simulink model "SF015A_WhlImbRejctn"  (R2013b)
settings: Solver=FixedStepDiscrete  SolverMode=SingleTasking  StartTime=0.0  StopTime=1  FixedStep=0.002  RelTol=1e-3
values from neighbouring files (symbols this model uses):
  ACTIVBANDMAX_ULS_U32 = DataDict.Constant    [SF015A_WhlImbRejctn_DataDict.m]
  ADAPVFILMAX_ULS_F32 = DataDict.Constant    [SF015A_WhlImbRejctn_DataDict.m]
  ARCHGLBPRM_180OVERPI_ULS_F32 = DataDict.Constant    [SF015A_WhlImbRejctn_DataDict.m]
  ARCHGLBPRM_2MILLISEC_SEC_F32 = DataDict.Constant    [SF015A_WhlImbRejctn_DataDict.m]
  ARCHGLBPRM_2PI_ULS_F32 = DataDict.Constant    [SF015A_WhlImbRejctn_DataDict.m]
  ARCHGLBPRM_FLOATZEROTHD_ULS_F32 = DataDict.Constant    [SF015A_WhlImbRejctn_DataDict.m]
  ARCHGLBPRM_PI_ULS_F32 = DataDict.Constant    [SF015A_WhlImbRejctn_DataDict.m]
  ARCHGLBPRM_PIOVER180_ULS_F32 = DataDict.Constant    [SF015A_WhlImbRejctn_DataDict.m]
  ARCHGLBPRM_PIOVER2_ULS_F32 = DataDict.Constant    [SF015A_WhlImbRejctn_DataDict.m]
  CALMINSPERCOUNT_ULS_F32 = DataDict.Constant    [SF015A_WhlImbRejctn_DataDict.m]
  DURATIONDISABLE_CNT_U16 = DataDict.Constant    [SF015A_WhlImbRejctn_DataDict.m]
  FILTWHLSPDMAX_MOTRADPERSEC_F32 = DataDict.Constant    [SF015A_WhlImbRejctn_DataDict.m]
  MICROSECTOMILLISEC_ULS_F32 = DataDict.Constant    [SF015A_WhlImbRejctn_DataDict.m]
  MINSTOMILLISEC_ULS_F32 = DataDict.Constant    [SF015A_WhlImbRejctn_DataDict.m]
  NINETY_ULS_F32 = DataDict.Constant    [SF015A_WhlImbRejctn_DataDict.m]
  NODEBSTEP_CNT_U16 = DataDict.Constant    [SF015A_WhlImbRejctn_DataDict.m]
  NROFDLY_CNT_U08 = DataDict.Constant    [SF015A_WhlImbRejctn_DataDict.m]
  ONEHALF_ULS_F32 = DataDict.Constant    [SF015A_WhlImbRejctn_DataDict.m]
  ONEHUNDRED_ULS_F32 = DataDict.Constant    [SF015A_WhlImbRejctn_DataDict.m]
  ONEOVRTHREE_ULS_F32 = DataDict.Constant    [SF015A_WhlImbRejctn_DataDict.m]
  ONEOVRTWENTY_ULS_F32 = DataDict.Constant    [SF015A_WhlImbRejctn_DataDict.m]
  ONETHOUSAND_ULS_F32 = DataDict.Constant    [SF015A_WhlImbRejctn_DataDict.m]
  PEAKMAX_ULS_F32 = DataDict.Constant    [SF015A_WhlImbRejctn_DataDict.m]
  PEAKMIN_ULS_F32 = DataDict.Constant    [SF015A_WhlImbRejctn_DataDict.m]
  PHAADJMAX_ULS_F32 = DataDict.Constant    [SF015A_WhlImbRejctn_DataDict.m]
  PITIMESSAMPLETIME_ULS_F32 = DataDict.Constant    [SF015A_WhlImbRejctn_DataDict.m]
  STOREDMINSPERCOUNT_ULS_F32 = DataDict.Constant    [SF015A_WhlImbRejctn_DataDict.m]
  TWO_ULS_F32 = DataDict.Constant    [SF015A_WhlImbRejctn_DataDict.m]
  TWOOVRTHREE_ULS_F32 = DataDict.Constant    [SF015A_WhlImbRejctn_DataDict.m]
  WhlImbRejctnAdpvFac = DataDict.Calibration    [SF015A_WhlImbRejctn_DataDict.m]
  WhlImbRejctnAutScaEna = DataDict.Calibration    [SF015A_WhlImbRejctn_DataDict.m]
  WhlImbRejctnAutScaTar = DataDict.Calibration    [SF015A_WhlImbRejctn_DataDict.m]
  WhlImbRejctnCurrMgnSlewPerLoop = DataDict.Calibration    [SF015A_WhlImbRejctn_DataDict.m]
  WhlImbRejctnDcTrendFltRcvryDly = DataDict.Calibration    [SF015A_WhlImbRejctn_DataDict.m]
  WhlImbRejctnDcTrendFltRcvryNegStep = DataDict.Calibration    [SF015A_WhlImbRejctn_DataDict.m]
  WhlImbRejctnDcTrendFltRcvryPosStep = DataDict.Calibration    [SF015A_WhlImbRejctn_DataDict.m]
  WhlImbRejctnDcTrendFltRcvryThd = DataDict.Calibration    [SF015A_WhlImbRejctn_DataDict.m]
  WhlImbRejctnDcTrendTh2Tq = DataDict.Calibration    [SF015A_WhlImbRejctn_DataDict.m]
  WhlImbRejctnDcTrendThTq = DataDict.Calibration    [SF015A_WhlImbRejctn_DataDict.m]
  WhlImbRejctnDcTrendTi2Sec = DataDict.Calibration    [SF015A_WhlImbRejctn_DataDict.m]
  WhlImbRejctnDcTrendTiSec = DataDict.Calibration    [SF015A_WhlImbRejctn_DataDict.m]
  WhlImbRejctnEnaSlewPerLoop = DataDict.Calibration    [SF015A_WhlImbRejctn_DataDict.m]
  WhlImbRejctnFctEna = DataDict.Calibration    [SF015A_WhlImbRejctn_DataDict.m]
  WhlImbRejctnFrqDiagcAmpThd = DataDict.Calibration    [SF015A_WhlImbRejctn_DataDict.m]
  WhlImbRejctnFrqDiagcEna = DataDict.Calibration    [SF015A_WhlImbRejctn_DataDict.m]
  WhlImbRejctnFrqDiagcFltRcvryDly = DataDict.Calibration    [SF015A_WhlImbRejctn_DataDict.m]
  WhlImbRejctnFrqDiagcFltRcvryNegStep = DataDict.Calibration    [SF015A_WhlImbRejctn_DataDict.m]
  WhlImbRejctnFrqDiagcFltRcvryPosStep = DataDict.Calibration    [SF015A_WhlImbRejctn_DataDict.m]
  WhlImbRejctnFrqDiagcFltRcvryThd = DataDict.Calibration    [SF015A_WhlImbRejctn_DataDict.m]
  WhlImbRejctnFrqDiagcThd = DataDict.Calibration    [SF015A_WhlImbRejctn_DataDict.m]
  WhlImbRejctnFrqDiagcTout = DataDict.Calibration    [SF015A_WhlImbRejctn_DataDict.m]
  WhlImbRejctnFrqDiagcUgrPoleMgn = DataDict.Calibration    [SF015A_WhlImbRejctn_DataDict.m]
  WhlImbRejctnFrqScaTblX = DataDict.Calibration    [SF015A_WhlImbRejctn_DataDict.m]
  WhlImbRejctnMaxDurn = DataDict.Calibration    [SF015A_WhlImbRejctn_DataDict.m]
  WhlImbRejctnMaxMgn = DataDict.Calibration    [SF015A_WhlImbRejctn_DataDict.m]
  WhlImbRejctnMaxMgnFltNegStep = DataDict.Calibration    [SF015A_WhlImbRejctn_DataDict.m]
  WhlImbRejctnMaxMgnFltPosStep = DataDict.Calibration    [SF015A_WhlImbRejctn_DataDict.m]
  WhlImbRejctnMaxMgnFltRcvryDly = DataDict.Calibration    [SF015A_WhlImbRejctn_DataDict.m]
  WhlImbRejctnMaxMgnFltRcvryNegStep = DataDict.Calibration    [SF015A_WhlImbRejctn_DataDict.m]
  WhlImbRejctnMaxMgnFltRcvryPosStep = DataDict.Calibration    [SF015A_WhlImbRejctn_DataDict.m]
  WhlImbRejctnMaxMgnFltRcvryThd = DataDict.Calibration    [SF015A_WhlImbRejctn_DataDict.m]
  WhlImbRejctnMaxMgnFltThd = DataDict.Calibration    [SF015A_WhlImbRejctn_DataDict.m]
  WhlImbRejctnMgnEstimnDeltaSca = DataDict.Calibration    [SF015A_WhlImbRejctn_DataDict.m]
  WhlImbRejctnMgnEstimnDiThd = DataDict.Calibration    [SF015A_WhlImbRejctn_DataDict.m]
  WhlImbRejctnMgnEstimnEnaThd = DataDict.Calibration    [SF015A_WhlImbRejctn_DataDict.m]
  WhlImbRejctnMgnEstimnFrq = DataDict.Calibration    [SF015A_WhlImbRejctn_DataDict.m]
  WhlImbRejctnMgnEstimnFrqDelta = DataDict.Calibration    [SF015A_WhlImbRejctn_DataDict.m]
  WhlImbRejctnMgnEstimnLeak = DataDict.Calibration    [SF015A_WhlImbRejctn_DataDict.m]
  WhlImbRejctnRampDwnTi = DataDict.Calibration    [SF015A_WhlImbRejctn_DataDict.m]
  WhlImbRejctnScaCncl = DataDict.Calibration    [SF015A_WhlImbRejctn_DataDict.m]
  WhlImbRejctnUgrPoleMgn = DataDict.Calibration    [SF015A_WhlImbRejctn_DataDict.m]
  WhlImbRejctnVehSpdEna = DataDict.Calibration    [SF015A_WhlImbRejctn_DataDict.m]
  WhlImbRejctnWhlSpdCorrlnFltRcvryDly = DataDict.Calibration    [SF015A_WhlImbRejctn_DataDict.m]
  WhlImbRejctnWhlSpdCorrlnFltRcvryNegStep = DataDict.Calibration    [SF015A_WhlImbRejctn_DataDict.m]
  WhlImbRejctnWhlSpdCorrlnFltRcvryPosStep = DataDict.Calibration    [SF015A_WhlImbRejctn_DataDict.m]
  WhlImbRejctnWhlSpdCorrlnFltRcvryThd = DataDict.Calibration    [SF015A_WhlImbRejctn_DataDict.m]
  WhlImbRejctnWhlSpdCorrlnThd = DataDict.Calibration    [SF015A_WhlImbRejctn_DataDict.m]
  WhlImbRejctnWhlSpdCorrlnTi = DataDict.Calibration    [SF015A_WhlImbRejctn_DataDict.m]
  WIRCMDMAX_MOTNWTMTR_F32 = DataDict.Constant    [SF015A_WhlImbRejctn_DataDict.m]
  ZERO_ULS_F32 = DataDict.Constant    [SF015A_WhlImbRejctn_DataDict.m]
undefined symbols (not defined in the file or in its folder): Cntr, NtcNr1, NvmGetErrSts1, SigQlfr1, Sts, SysSt1
libraries: simulink x32, FixdToFloat x32, Fil x20, NxtrLim x15, NxtrNvM x12, NxtrAbslt x8, NxtrMath x7, NxtrMax x6, NxtrMin x4, FloatToFixd x2, LnrIntrpn x2, NxtrSign x1
(part 3 of 12)

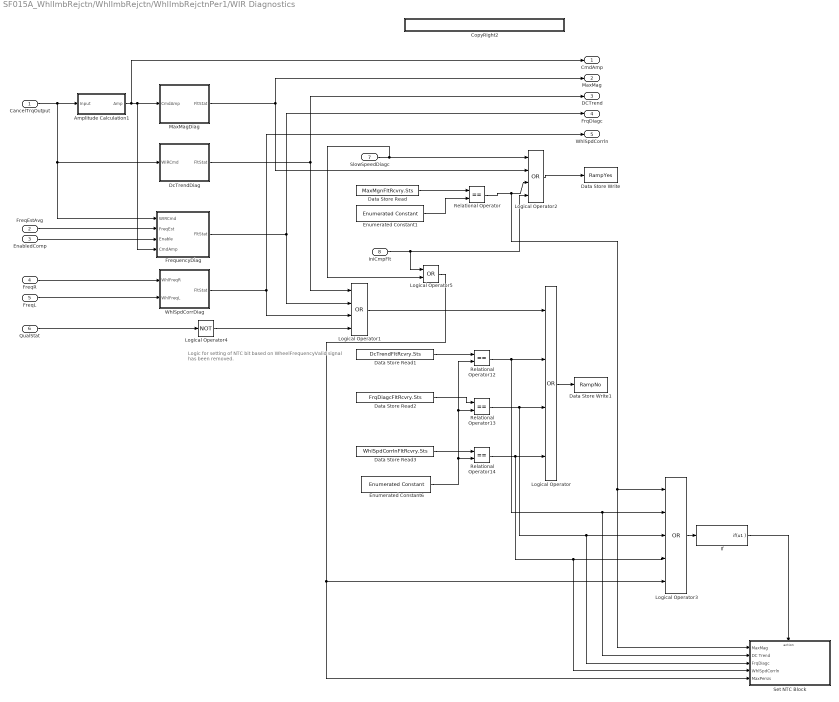
== system SF015A_WhlImbRejctn/WhlImbRejctn/WhlImbRejctnPer1/WIR Diagnostics ==
  note: Logic for setting of NTC bit based on WheelFrequencyValid
      | signal has been removed.
  CancelTrqOutput : Inport
  FreqEstAvg : Inport  Port=2
  EnabledComp : Inport  Port=3
  FreqR : Inport  Port=4
  FreqL : Inport  Port=5
  QualStat : Inport  Port=6
  "SlowSpeedDiagc " : Inport  Port=7
  IniCmpFlt : Inport  Port=8
  Amplitude Calculation1 : Subsystem
  CopyRight2 : Subsystem  Description=|  mask(Copyright Information){none=on}
      | Copyright info block.                                               
      |                                                                     
      | Place copyright information at the top of every subsystem in design.
      mask prompts: none "No parameters"
      mask help: Place copyright information at the top of every subsystem in design.
      mask Display:
      | NxtrConf = 'Nexteer Confidential';
      | 
      | sys = bdroot; %handle for the current model ("system")
      | first = get_param(sys,'Created');
      | first = first(end-3:end);  %year is last four digits
      | 
      | last = get_param(sys,'LastModifiedDate');
      | if isempty(last)
      |     last = datestr(now,'yyyy');
      | else
      |     last = last(end-3:end);
      | end
      | 
      | if strcmp(first,last)
      |     fprintf('%s -- Copyright %s Nexteer',NxtrConf,first)
      | else
      |     fprintf('%s -- %s%s- %s Nexteer',NxtrConf,char(169),first,last)
      | end
  Data Store Read : DataStoreRead  DataStoreName=MaxMgnFltRcvry  DataStoreElements=MaxMgnFltRcvry.Sts
  Data Store Read1 : DataStoreRead  DataStoreName=DcTrendFltRcvry  DataStoreElements=DcTrendFltRcvry.Sts
  Data Store Read2 : DataStoreRead  DataStoreName=FrqDiagcFltRcvry  DataStoreElements=FrqDiagcFltRcvry.Sts
  Data Store Read3 : DataStoreRead  DataStoreName=WhlSpdCorrlnFltRcvry  DataStoreElements=WhlSpdCorrlnFltRcvry.Sts
  Data Store Write : DataStoreWrite  DataStoreName=RampYes
  Data Store Write1 : DataStoreWrite  DataStoreName=RampNo
  DcTrendDiag : Subsystem
  Enumerated Constant1 : simulink/Sources/Enumerated Constant  OutDataTypeStr=Enum: SigQlfr1  Value=SigQlfr1.SIGQLFR_FAILD  SampleTime=inf
  Enumerated Constant6 : simulink/Sources/Enumerated Constant  OutDataTypeStr=Enum: SigQlfr1  Value=SigQlfr1.SIGQLFR_FAILD  SampleTime=inf
  FrequencyDiag : Subsystem
  If : If  IfExpression=u1  ShowElse=off
  Logical Operator : Logic  Operator=OR  Inputs=4  AllPortsSameDT=off  OutDataTypeStr=boolean
  Logical Operator1 : Logic  Operator=OR  Inputs=4  AllPortsSameDT=off  OutDataTypeStr=boolean
  Logical Operator2 : Logic  Operator=OR  Inputs=4  AllPortsSameDT=off  OutDataTypeStr=boolean
  Logical Operator3 : Logic  Operator=OR  Inputs=5  AllPortsSameDT=off  OutDataTypeStr=boolean
  Logical Operator4 : Logic  Operator=NOT  AllPortsSameDT=off  OutDataTypeStr=boolean
  Logical Operator5 : Logic  Operator=OR  AllPortsSameDT=off  OutDataTypeStr=boolean
  MaxMagDiag : Subsystem
  Relational Operator{,12..14} (4 alike) : RelationalOperator  Operator===  OutDataTypeStr=boolean
  Set NTC Block : Subsystem  TreatAsAtomicUnit=on
  WhlSpdCorrDiag : Subsystem
  CmdAmp : Outport
  MaxMag : Outport  Port=2
  DCTrend : Outport  Port=3
  FrqDiagc : Outport  Port=4
  WhlSpdCorrln : Outport  Port=5
  wires:
  CancelTrqOutput/1 -> Amplitude Calculation1/1(Input), FrequencyDiag/1(WIRCmd), DcTrendDiag/1(WIRCmd)
  EnabledComp/1 -> FrequencyDiag/3(Enable)
  FreqEstAvg/1 -> FrequencyDiag/2(FreqEst)
  FreqR/1 -> WhlSpdCorrDiag/1(WhlFreqR)
  FreqL/1 -> WhlSpdCorrDiag/2(WhlFreqL)
  DcTrendDiag/1(FltStat) -> DCTrend/1, Logical Operator1/1
  MaxMagDiag/1(FltStat) -> MaxMag/1, Logical Operator2/2
  FrequencyDiag/1(FltStat) -> FrqDiagc/1, Logical Operator1/2
  WhlSpdCorrDiag/1(FltStat) -> WhlSpdCorrln/1, Logical Operator1/3
  Amplitude Calculation1/1(Amp) -> CmdAmp/1, MaxMagDiag/1(CmdAmp), FrequencyDiag/4(CmdAmp)
  Relational Operator12/1 -> Logical Operator/2, Set NTC Block/2(DC Trend), Logical Operator3/2
  Relational Operator14/1 -> Logical Operator3/4, Set NTC Block/4(WhlSpdCorrln), Logical Operator/4
  Enumerated Constant6/1 -> Relational Operator12/2, Relational Operator13/2, Relational Operator14/2
  Logical Operator1/1 -> Logical Operator/1
  Logical Operator2/1 -> Data Store Write/1
  "SlowSpeedDiagc "/1 -> Logical Operator5/2, Logical Operator2/1
  Data Store Read/1 -> Relational Operator/1
  Enumerated Constant1/1 -> Relational Operator/2
  Relational Operator/1 -> Set NTC Block/1(MaxMag), Logical Operator3/1, Logical Operator2/3
  Data Store Read1/1 -> Relational Operator12/1
  Data Store Read3/1 -> Relational Operator14/1
  Data Store Read2/1 -> Relational Operator13/1
  Logical Operator3/1 -> If/1
  If/1 -> Set NTC Block/Action
  Logical Operator/1 -> Data Store Write1/1
  Relational Operator13/1 -> Logical Operator3/3, Set NTC Block/3(FrqDiagc), Logical Operator/3
  QualStat/1 -> Logical Operator4/1
  Logical Operator4/1 -> Logical Operator1/4
  IniCmpFlt/1 -> Logical Operator5/1, Logical Operator2/4
  Logical Operator5/1 -> Logical Operator3/5, Set NTC Block/5(MaxPersis)

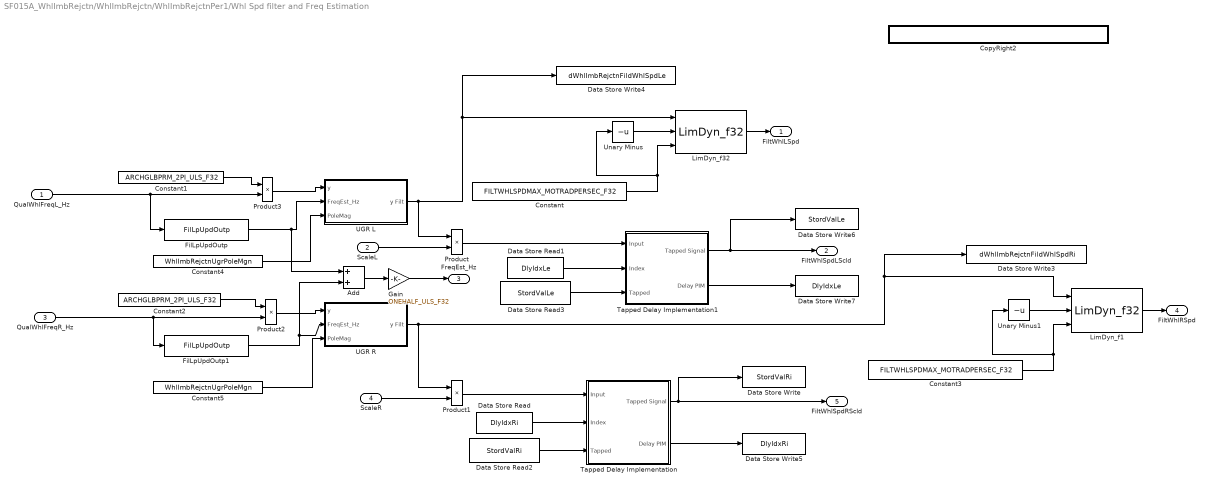
== system SF015A_WhlImbRejctn/WhlImbRejctn/WhlImbRejctnPer1/Whl Spd filter and Freq Estimation ==
  QualWhlFreqL_Hz : Inport
  ScaleL : Inport  Port=2
  QualWhlFreqR_Hz : Inport  Port=3
  ScaleR : Inport  Port=4
  Add : Sum
  Constant : Constant  Value=FILTWHLSPDMAX_MOTRADPERSEC_F32
  Constant1 : Constant  Value=ARCHGLBPRM_2PI_ULS_F32
  Constant2 : Constant  Value=ARCHGLBPRM_2PI_ULS_F32
  Constant3 : Constant  Value=FILTWHLSPDMAX_MOTRADPERSEC_F32
  Constant4 : Constant  Value=WhlImbRejctnUgrPoleMgn
  Constant5 : Constant  Value=WhlImbRejctnUgrPoleMgn
  CopyRight2 : Subsystem  Description=|  mask(Copyright Information){none=on}
      | Copyright info block.                                               
      |                                                                     
      | Place copyright information at the top of every subsystem in design.
      mask prompts: none "No parameters"
      mask help: Place copyright information at the top of every subsystem in design.
      mask Display:
      | NxtrConf = 'Nexteer Confidential';
      | 
      | sys = bdroot; %handle for the current model ("system")
      | first = get_param(sys,'Created');
      | first = first(end-3:end);  %year is last four digits
      | 
      | last = get_param(sys,'LastModifiedDate');
      | if isempty(last)
      |     last = datestr(now,'yyyy');
      | else
      |     last = last(end-3:end);
      | end
      | 
      | if strcmp(first,last)
      |     fprintf('%s -- Copyright %s Nexteer',NxtrConf,first)
      | else
      |     fprintf('%s -- %s%s- %s Nexteer',NxtrConf,char(169),first,last)
      | end
  Data Store Read : DataStoreRead  DataStoreName=DlyIdxRi
  Data Store Read1 : DataStoreRead  DataStoreName=DlyIdxLe
  Data Store Read2 : DataStoreRead  DataStoreName=StordValRi
  Data Store Read3 : DataStoreRead  DataStoreName=StordValLe
  Data Store Write : DataStoreWrite  DataStoreName=StordValRi
  Data Store Write3 : DataStoreWrite  DataStoreName=dWhlImbRejctnFildWhlSpdRi
  Data Store Write4 : DataStoreWrite  DataStoreName=dWhlImbRejctnFildWhlSpdLe
  Data Store Write5 : DataStoreWrite  DataStoreName=DlyIdxRi
  Data Store Write6 : DataStoreWrite  DataStoreName=StordValLe
  Data Store Write7 : DataStoreWrite  DataStoreName=DlyIdxLe
  FilLpUpdOutp : Fil/FilLpUpdOutp  StVar=WhlSpdLeLpFil
      settings: AttributesFormatString=StVar: %<StVar>
  FilLpUpdOutp1 : Fil/FilLpUpdOutp  StVar=WhlSpdRiLpFil
      settings: AttributesFormatString=StVar: %<StVar>
  Gain : Gain  Gain=ONEHALF_ULS_F32
  LimDyn_f1 : NxtrLim/LimDyn_f32
  LimDyn_f32 : NxtrLim/LimDyn_f32
  Product{,1..3} (4 alike) : Product
  Tapped Delay Implementation : Subsystem  TreatAsAtomicUnit=on
  Tapped Delay Implementation1 : Subsystem  TreatAsAtomicUnit=on
  UGR L : Subsystem
  UGR R : Subsystem
  Unary Minus : UnaryMinus
  Unary Minus1 : UnaryMinus
  FiltWhlLSpd : Outport
  FiltWhlSpdLScld : Outport  Port=2
  FreqEst_Hz : Outport  Port=3
  FiltWhlRSpd : Outport  Port=4
  FiltWhlSpdRScld : Outport  Port=5
  wires:
  UGR L/1(y Filt) -> Product/1, LimDyn_f32/1, Data Store Write4/1
  FilLpUpdOutp/1 -> Add/1, UGR L/2(FreqEst_Hz)
  QualWhlFreqL_Hz/1 -> FilLpUpdOutp/1, Product3/2
  Product/1 -> Tapped Delay Implementation1/1(Input)
  ScaleL/1 -> Product/2
  Constant1/1 -> Product3/1
  Product3/1 -> UGR L/1(y)
  UGR R/1(y Filt) -> Product1/1, Data Store Write3/1, LimDyn_f1/1
  FilLpUpdOutp1/1 -> UGR R/2(FreqEst_Hz), Add/2
  QualWhlFreqR_Hz/1 -> FilLpUpdOutp1/1, Product2/2
  Product1/1 -> Tapped Delay Implementation/1(Input)
  Constant2/1 -> Product2/1
  Product2/1 -> UGR R/1(y)
  ScaleR/1 -> Product1/2
  Add/1 -> Gain/1
  Gain/1 -> FreqEst_Hz/1
  Data Store Read/1 -> Tapped Delay Implementation/2(Index)
  Data Store Read2/1 -> Tapped Delay Implementation/3(Tapped)
  Tapped Delay Implementation/1(Tapped Signal) -> Data Store Write/1, FiltWhlSpdRScld/1
  Tapped Delay Implementation/2(Delay PIM) -> Data Store Write5/1
  Tapped Delay Implementation1/1(Tapped Signal) -> Data Store Write6/1, FiltWhlSpdLScld/1
  Tapped Delay Implementation1/2(Delay PIM) -> Data Store Write7/1
  Data Store Read1/1 -> Tapped Delay Implementation1/2(Index)
  Data Store Read3/1 -> Tapped Delay Implementation1/3(Tapped)
  LimDyn_f32/1 -> FiltWhlLSpd/1
  Constant/1 -> Unary Minus/1, LimDyn_f32/3
  Unary Minus/1 -> LimDyn_f32/2
  LimDyn_f1/1 -> FiltWhlRSpd/1
  Constant3/1 -> Unary Minus1/1, LimDyn_f1/3
  Unary Minus1/1 -> LimDyn_f1/2
  Constant4/1 -> UGR L/3(PoleMag)
  Constant5/1 -> UGR R/3(PoleMag)

== system SF015A_WhlImbRejctn/WhlImbRejctn/WhlImbRejctnPer2/CopyRight2 ==

== system SF015A_WhlImbRejctn/WhlImbRejctn/WhlImbRejctnPer2/Flt Recovery- DC Trend ==
  FltStatIn : Inport
  FltRecDly : Inport  Port=2
  Constant : Constant  Value=MINSTOMILLISEC_ULS_F32
  CopyRight2 : Subsystem  Description=|  mask(Copyright Information){none=on}
      | Copyright info block.                                               
      |                                                                     
      | Place copyright information at the top of every subsystem in design.
      mask prompts: none "No parameters"
      mask help: Place copyright information at the top of every subsystem in design.
      mask Display:
      | NxtrConf = 'Nexteer Confidential';
      | 
      | sys = bdroot; %handle for the current model ("system")
      | first = get_param(sys,'Created');
      | first = first(end-3:end);  %year is last four digits
      | 
      | last = get_param(sys,'LastModifiedDate');
      | if isempty(last)
      |     last = datestr(now,'yyyy');
      | else
      |     last = last(end-3:end);
      | end
      | 
      | if strcmp(first,last)
      |     fprintf('%s -- Copyright %s Nexteer',NxtrConf,first)
      | else
      |     fprintf('%s -- %s%s- %s Nexteer',NxtrConf,char(169),first,last)
      | end
  Data Store Read : DataStoreRead  Priority=1  DataStoreName=DcTrendFltRcvry
      settings: AttributesFormatString=Priority:%<Priority>
  Data Store Write1 : DataStoreWrite  Priority=2  DataStoreName=DcTrendFltRcvry
      settings: AttributesFormatString=Priority:%<Priority>
  Divide : Product  Inputs=**
  ElapsedTime1 : Subsystem  TreatAsAtomicUnit=on
  Relational Operator4 : RelationalOperator  OutDataTypeStr=boolean
  Update Fault Status : Subsystem  TreatAsAtomicUnit=on
  wires:
  ElapsedTime1/1(ElapsedTime) -> Relational Operator4/1
  FltStatIn/1 -> ElapsedTime1/1(FltStsTrue)
  FltRecDly/1 -> Divide/1
  Relational Operator4/1 -> Update Fault Status/2(Status)
  Data Store Read/1 -> Update Fault Status/1(Structvar)
  Update Fault Status/1(Structvar_out) -> Data Store Write1/1
  Divide/1 -> Relational Operator4/2
  Constant/1 -> Divide/2

== system SF015A_WhlImbRejctn/WhlImbRejctn/WhlImbRejctnPer2/Flt Recovery- Freq Diag ==
  FltStatIn : Inport
  FltRecDly : Inport  Port=2
  Constant : Constant  Value=MINSTOMILLISEC_ULS_F32
  CopyRight2 : Subsystem  Description=|  mask(Copyright Information){none=on}
      | Copyright info block.                                               
      |                                                                     
      | Place copyright information at the top of every subsystem in design.
      mask prompts: none "No parameters"
      mask help: Place copyright information at the top of every subsystem in design.
      mask Display:
      | NxtrConf = 'Nexteer Confidential';
      | 
      | sys = bdroot; %handle for the current model ("system")
      | first = get_param(sys,'Created');
      | first = first(end-3:end);  %year is last four digits
      | 
      | last = get_param(sys,'LastModifiedDate');
      | if isempty(last)
      |     last = datestr(now,'yyyy');
      | else
      |     last = last(end-3:end);
      | end
      | 
      | if strcmp(first,last)
      |     fprintf('%s -- Copyright %s Nexteer',NxtrConf,first)
      | else
      |     fprintf('%s -- %s%s- %s Nexteer',NxtrConf,char(169),first,last)
      | end
  Data Store Read : DataStoreRead  Priority=1  DataStoreName=FrqDiagcFltRcvry
      settings: AttributesFormatString=Priority:%<Priority>
  Data Store Write1 : DataStoreWrite  Priority=2  DataStoreName=FrqDiagcFltRcvry
      settings: AttributesFormatString=Priority:%<Priority>
  Divide : Product  Inputs=**
  ElapsedTime1 : Subsystem  TreatAsAtomicUnit=on
  Relational Operator4 : RelationalOperator  OutDataTypeStr=boolean
  Update Fault Status : Subsystem  TreatAsAtomicUnit=on
  wires:
  ElapsedTime1/1(ElapsedTime) -> Relational Operator4/1
  FltStatIn/1 -> ElapsedTime1/1(FltStsTrue)
  FltRecDly/1 -> Divide/1
  Data Store Read/1 -> Update Fault Status/1(Structvar)
  Update Fault Status/1(Structvar_out) -> Data Store Write1/1
  Relational Operator4/1 -> Update Fault Status/2(Status)
  Divide/1 -> Relational Operator4/2
  Constant/1 -> Divide/2

== system SF015A_WhlImbRejctn/WhlImbRejctn/WhlImbRejctnPer2/Flt Recovery- Max Mag ==
  FltStatIn : Inport
  FltRecDly : Inport  Port=2
  Constant : Constant  Value=MINSTOMILLISEC_ULS_F32
  CopyRight2 : Subsystem  Description=|  mask(Copyright Information){none=on}
      | Copyright info block.                                               
      |                                                                     
      | Place copyright information at the top of every subsystem in design.
      mask prompts: none "No parameters"
      mask help: Place copyright information at the top of every subsystem in design.
      mask Display:
      | NxtrConf = 'Nexteer Confidential';
      | 
      | sys = bdroot; %handle for the current model ("system")
      | first = get_param(sys,'Created');
      | first = first(end-3:end);  %year is last four digits
      | 
      | last = get_param(sys,'LastModifiedDate');
      | if isempty(last)
      |     last = datestr(now,'yyyy');
      | else
      |     last = last(end-3:end);
      | end
      | 
      | if strcmp(first,last)
      |     fprintf('%s -- Copyright %s Nexteer',NxtrConf,first)
      | else
      |     fprintf('%s -- %s%s- %s Nexteer',NxtrConf,char(169),first,last)
      | end
  Data Store Read : DataStoreRead  Priority=1  DataStoreName=MaxMgnFltRcvry
      settings: AttributesFormatString=Priority:%<Priority>
  Data Store Write1 : DataStoreWrite  Priority=2  DataStoreName=MaxMgnFltRcvry
      settings: AttributesFormatString=Priority:%<Priority>
  Divide : Product  Inputs=**
  ElapsedTime1 : Subsystem  TreatAsAtomicUnit=on
  Relational Operator4 : RelationalOperator  OutDataTypeStr=boolean
  Update Fault Status : Subsystem  TreatAsAtomicUnit=on
  wires:
  ElapsedTime1/1(ElapsedTime) -> Relational Operator4/1
  FltStatIn/1 -> ElapsedTime1/1(FltStsTrue)
  FltRecDly/1 -> Divide/1
  Relational Operator4/1 -> Update Fault Status/2(Status)
  Data Store Read/1 -> Update Fault Status/1(Structvar)
  Update Fault Status/1(Structvar_out) -> Data Store Write1/1
  Divide/1 -> Relational Operator4/2
  Constant/1 -> Divide/2

== system SF015A_WhlImbRejctn/WhlImbRejctn/WhlImbRejctnPer2/Flt Recovery- WhlSpdCorr Diag ==
  FltStatIn : Inport
  FltRecDly : Inport  Port=2
  Constant : Constant  Value=MINSTOMILLISEC_ULS_F32
  CopyRight2 : Subsystem  Description=|  mask(Copyright Information){none=on}
      | Copyright info block.                                               
      |                                                                     
      | Place copyright information at the top of every subsystem in design.
      mask prompts: none "No parameters"
      mask help: Place copyright information at the top of every subsystem in design.
      mask Display:
      | NxtrConf = 'Nexteer Confidential';
      | 
      | sys = bdroot; %handle for the current model ("system")
      | first = get_param(sys,'Created');
      | first = first(end-3:end);  %year is last four digits
      | 
      | last = get_param(sys,'LastModifiedDate');
      | if isempty(last)
      |     last = datestr(now,'yyyy');
      | else
      |     last = last(end-3:end);
      | end
      | 
      | if strcmp(first,last)
      |     fprintf('%s -- Copyright %s Nexteer',NxtrConf,first)
      | else
      |     fprintf('%s -- %s%s- %s Nexteer',NxtrConf,char(169),first,last)
      | end
  Data Store Read : DataStoreRead  Priority=1  DataStoreName=WhlSpdCorrlnFltRcvry
      settings: AttributesFormatString=Priority:%<Priority>
  Data Store Write1 : DataStoreWrite  Priority=2  DataStoreName=WhlSpdCorrlnFltRcvry
      settings: AttributesFormatString=Priority:%<Priority>
  Divide : Product  Inputs=**
  ElapsedTime1 : Subsystem  TreatAsAtomicUnit=on
  Relational Operator4 : RelationalOperator  OutDataTypeStr=boolean
  Update Fault Status : Subsystem  TreatAsAtomicUnit=on
  wires:
  ElapsedTime1/1(ElapsedTime) -> Relational Operator4/1
  FltStatIn/1 -> ElapsedTime1/1(FltStsTrue)
  FltRecDly/1 -> Divide/1
  Data Store Read/1 -> Update Fault Status/1(Structvar)
  Update Fault Status/1(Structvar_out) -> Data Store Write1/1
  Relational Operator4/1 -> Update Fault Status/2(Status)
  Divide/1 -> Relational Operator4/2
  Constant/1 -> Divide/2

== system SF015A_WhlImbRejctn/WhlImbRejctn/WhlImbRejctnPer2/WIR Low Speed Diagnostics ==
  CmdAmp : Inport
  CopyRight2 : Subsystem  Description=|  mask(Copyright Information){none=on}
      | Copyright info block.                                               
      |                                                                     
      | Place copyright information at the top of every subsystem in design.
      mask prompts: none "No parameters"
      mask help: Place copyright information at the top of every subsystem in design.
      mask Display:
      | NxtrConf = 'Nexteer Confidential';
      | 
      | sys = bdroot; %handle for the current model ("system")
      | first = get_param(sys,'Created');
      | first = first(end-3:end);  %year is last four digits
      | 
      | last = get_param(sys,'LastModifiedDate');
      | if isempty(last)
      |     last = datestr(now,'yyyy');
      | else
      |     last = last(end-3:end);
      | end
      | 
      | if strcmp(first,last)
      |     fprintf('%s -- Copyright %s Nexteer',NxtrConf,first)
      | else
      |     fprintf('%s -- %s%s- %s Nexteer',NxtrConf,char(169),first,last)
      | end
  MaxPersisDiag : Subsystem
  WIRFltStatus_SlowSpeed : Outport
  wires:
  CmdAmp/1 -> MaxPersisDiag/1(CmdAmp)
  MaxPersisDiag/1(MaxPersistence_fault) -> WIRFltStatus_SlowSpeed/1

== system SF015A_WhlImbRejctn/WhlImbRejctn/WhlImbRejctnInit1/Check NVM Data/CheckCompPersistence ==
  ActiveBand1 : Inport
  ActiveBand2 : Inport  Port=2
  ActiveBand3 : Inport  Port=3
  Constant1 : Constant  Value=WhlImbRejctnMaxDurn
  Constant15 : Constant  Value=0  OutDataTypeStr=boolean
  Constant3 : Constant  Value=DURATIONDISABLE_CNT_U16
  CopyRight2 : Subsystem  Description=|  mask(Copyright Information){none=on}
      | Copyright info block.                                               
      |                                                                     
      | Place copyright information at the top of every subsystem in design.
      mask prompts: none "No parameters"
      mask help: Place copyright information at the top of every subsystem in design.
      mask Display:
      | NxtrConf = 'Nexteer Confidential';
      | 
      | sys = bdroot; %handle for the current model ("system")
      | first = get_param(sys,'Created');
      | first = first(end-3:end);  %year is last four digits
      | 
      | last = get_param(sys,'LastModifiedDate');
      | if isempty(last)
      |     last = datestr(now,'yyyy');
      | else
      |     last = last(end-3:end);
      | end
      | 
      | if strcmp(first,last)
      |     fprintf('%s -- Copyright %s Nexteer',NxtrConf,first)
      | else
      |     fprintf('%s -- %s%s- %s Nexteer',NxtrConf,char(169),first,last)
      | end
  Data Type Conversion1 : DataTypeConversion  OutDataTypeStr=boolean
  If1 : If  IfExpression=u1
  Merge5 : Merge
  NoFault : Subsystem  RequirementInfo={} %GIDa_ba94ca7d_ee6a_41fe_9637_ca38a72bc55f  TreatAsAtomicUnit=on
  Relational Operator1 : RelationalOperator  Operator=<=  OutDataTypeStr=boolean
  Subsystem : Subsystem
  Fault : Outport
  wires:
  Constant1/1 -> Relational Operator1/1
  Relational Operator1/1 -> If1/1
  Constant3/1 -> Relational Operator1/2
  If1/1 -> Subsystem/Action
  ActiveBand1/1 -> Subsystem/1(Band)
  ActiveBand2/1 -> Subsystem/2(Band2)
  ActiveBand3/1 -> Subsystem/3(Band3)
  Merge5/1 -> Fault/1
  Subsystem/1(Fault) -> Merge5/1
  Constant15/1 -> Data Type Conversion1/1
  NoFault/1(Output) -> Merge5/2
  If1/2 -> NoFault/Action
  Data Type Conversion1/1 -> NoFault/1(Input)

== system SF015A_WhlImbRejctn/WhlImbRejctn/WhlImbRejctnInit1/Check NVM Data/NvmNotVal ==
  Action Port : ActionPort  ActionType=then
  Constant : Constant  Value=ZERO_ULS_F32
  CopyRight2 : Subsystem  Description=|  mask(Copyright Information){none=on}
      | Copyright info block.                                               
      |                                                                     
      | Place copyright information at the top of every subsystem in design.
      mask prompts: none "No parameters"
      mask help: Place copyright information at the top of every subsystem in design.
      mask Display:
      | NxtrConf = 'Nexteer Confidential';
      | 
      | sys = bdroot; %handle for the current model ("system")
      | first = get_param(sys,'Created');
      | if(isempty(first))
      |     first = datestr(now,'yyyy');
      | else
      |     first = first(end-3:end);  %year is last four digits
      | end
      | 
      | last = get_param(sys,'LastModifiedDate');
      | if isempty(last)
      |     last = datestr(now,'yyyy');
      | else
      |     last = last(end-3:end);
      | end
      | 
      | if strcmp(first,last)
      |     fprintf('%s -- Copyright %s Nexteer',NxtrConf,first)
      | else
      |     fprintf('%s -- %s%s- %s Nexteer',NxtrConf,char(169),first,last)
      | end
  Data Store Write : DataStoreWrite  DataStoreName=ActvCmpBand2
  Data Store Write1 : DataStoreWrite  DataStoreName=MaxCompPerc
  Data Store Write2 : DataStoreWrite  DataStoreName=ActvCmpBand3
  Data Store Write3 : DataStoreWrite  DataStoreName=ActvCmpBand1
  Data Store Write4 : DataStoreWrite  DataStoreName=RiPeakPrev
  Data Store Write5 : DataStoreWrite  DataStoreName=LePeakPrev
  Data Type Conversion : DataTypeConversion  OutDataTypeStr=uint32
  Data Type Conversion1 : DataTypeConversion  OutDataTypeStr=uint32
  Data Type Conversion2 : DataTypeConversion  OutDataTypeStr=uint32
  wires:
  Constant/1 -> Data Store Write4/1, Data Store Write5/1, Data Store Write1/1, Data Type Conversion2/1, Data Type Conversion1/1, Data Type Conversion/1
  Data Type Conversion/1 -> Data Store Write3/1
  Data Type Conversion1/1 -> Data Store Write/1
  Data Type Conversion2/1 -> Data Store Write2/1

== system SF015A_WhlImbRejctn/WhlImbRejctn/WhlImbRejctnInit1/Check NVM Data/ResetNVM ==
  Action Port : ActionPort  ActionType=then
  Constant : Constant  Value=ZERO_ULS_F32
  CopyRight2 : Subsystem  Description=|  mask(Copyright Information){none=on}
      | Copyright info block.                                               
      |                                                                     
      | Place copyright information at the top of every subsystem in design.
      mask prompts: none "No parameters"
      mask help: Place copyright information at the top of every subsystem in design.
      mask Display:
      | NxtrConf = 'Nexteer Confidential';
      | 
      | sys = bdroot; %handle for the current model ("system")
      | first = get_param(sys,'Created');
      | if(isempty(first))
      |     first = datestr(now,'yyyy');
      | else
      |     first = first(end-3:end);  %year is last four digits
      | end
      | 
      | last = get_param(sys,'LastModifiedDate');
      | if isempty(last)
      |     last = datestr(now,'yyyy');
      | else
      |     last = last(end-3:end);
      | end
      | 
      | if strcmp(first,last)
      |     fprintf('%s -- Copyright %s Nexteer',NxtrConf,first)
      | else
      |     fprintf('%s -- %s%s- %s Nexteer',NxtrConf,char(169),first,last)
      | end
  Data Store Write : DataStoreWrite  DataStoreName=ActvCmpBand2
  Data Store Write1 : DataStoreWrite  DataStoreName=MaxCompPerc
  Data Store Write2 : DataStoreWrite  DataStoreName=ActvCmpBand3
  Data Store Write3 : DataStoreWrite  DataStoreName=ActvCmpBand1
  Data Type Conversion : DataTypeConversion  OutDataTypeStr=uint32
  Data Type Conversion1 : DataTypeConversion  OutDataTypeStr=uint32
  Data Type Conversion2 : DataTypeConversion  OutDataTypeStr=uint32
  wires:
  Constant/1 -> Data Store Write1/1, Data Type Conversion2/1, Data Type Conversion1/1, Data Type Conversion/1
  Data Type Conversion/1 -> Data Store Write3/1
  Data Type Conversion1/1 -> Data Store Write/1
  Data Type Conversion2/1 -> Data Store Write2/1

== system SF015A_WhlImbRejctn/WhlImbRejctn/WhlImbRejctnInit1/Check NVM Data/ResetNVM1 ==
  Action Port : ActionPort  ActionType=then
  Constant : Constant  Value=ZERO_ULS_F32
  CopyRight2 : Subsystem  Description=|  mask(Copyright Information){none=on}
      | Copyright info block.                                               
      |                                                                     
      | Place copyright information at the top of every subsystem in design.
      mask prompts: none "No parameters"
      mask help: Place copyright information at the top of every subsystem in design.
      mask Display:
      | NxtrConf = 'Nexteer Confidential';
      | 
      | sys = bdroot; %handle for the current model ("system")
      | first = get_param(sys,'Created');
      | if(isempty(first))
      |     first = datestr(now,'yyyy');
      | else
      |     first = first(end-3:end);  %year is last four digits
      | end
      | 
      | last = get_param(sys,'LastModifiedDate');
      | if isempty(last)
      |     last = datestr(now,'yyyy');
      | else
      |     last = last(end-3:end);
      | end
      | 
      | if strcmp(first,last)
      |     fprintf('%s -- Copyright %s Nexteer',NxtrConf,first)
      | else
      |     fprintf('%s -- %s%s- %s Nexteer',NxtrConf,char(169),first,last)
      | end
  Data Store Write4 : DataStoreWrite  DataStoreName=RiPeakPrev
  Data Store Write5 : DataStoreWrite  DataStoreName=LePeakPrev
  wires:
  Constant/1 -> Data Store Write5/1, Data Store Write4/1

== system SF015A_WhlImbRejctn/WhlImbRejctn/WhlImbRejctnPer1/Active Rejection Command /Adaptive Filter - FloatingL ==
  note: Summation of
      | tapped delay elements
  Enable : Inport
  PrevEpsilon : Inport  Port=2
  AdaptiveMu : Inport  Port=3
  x Ref : Inport  Port=4
  Constant2 : Constant  Value=2  OutDataTypeStr=uint16
  Constant4 : Constant  Value=ADAPVFILMAX_ULS_F32
  Data Store Read1 : DataStoreRead  Priority=1  DataStoreName=LeStDlyUpd
      settings: AttributesFormatString=%<Priority>
  Data Store Read2 : DataStoreRead  Priority=1  DataStoreName=LeStVariUpd
      settings: AttributesFormatString=%<Priority>
  Data Store Write1 : DataStoreWrite  Priority=2  DataStoreName=LeStDlyUpd
      settings: AttributesFormatString=%<Priority>
  Data Store Write2 : DataStoreWrite  Priority=3  DataStoreName=LeStVariUpd
      settings: AttributesFormatString=%<Priority>
  Data Store Write3 : DataStoreWrite  DataStoreName=dWhlImbRejctnLMSqdOutLe
  LimDyn_f32 : NxtrLim/LimDyn_f32
  Product3 : Product  RndMeth=Nearest
  Product5 : Product  Inputs=3
  Product6 : Product  RndMeth=Nearest
  Product7 : Product
  Sum3 : Sum  Inputs=|++
  Sum4 : Sum  Inputs=+
  Unary Minus : UnaryMinus
  output : Outport
  wires:
  x Ref/1 -> Data Store Write1/1, Product7/2  "x_k"
  Product3/1 -> Product6/1  "Multiplier"
  [enable] -> Product3/1
  Data Store Read1/1 -> Product6/2  "x_k-1"
  Product7/1 -> Sum4/1
  Sum3/1 -> Data Store Write2/1, Product7/1  "W_k- xRefStaeVar"
  Product6/1 -> Sum3/1
  Product5/1 -> Product3/2
  AdaptiveMu/1 -> Product5/2
  PrevEpsilon/1 -> Product5/3  "eps_k-1"
  Constant2/1 -> Product5/1
  Enable/1 -> [enable]
  Constant4/1 -> Unary Minus/1, LimDyn_f32/3
  Unary Minus/1 -> LimDyn_f32/2
  Sum4/1 -> LimDyn_f32/1
  Data Store Read2/1 -> Sum3/2  "x_k-1"
  LimDyn_f32/1 -> Data Store Write3/1, output/1

== system SF015A_WhlImbRejctn/WhlImbRejctn/WhlImbRejctnPer1/Active Rejection Command /Adaptive Filter - FloatingR ==
  Enable : Inport
  PrevEpsilon : Inport  Port=2
  AdaptiveMu : Inport  Port=3
  x Ref : Inport  Port=4
  Constant2 : Constant  Value=2  OutDataTypeStr=uint16
  Constant4 : Constant  Value=ADAPVFILMAX_ULS_F32
  Data Store Read : DataStoreRead  DataStoreName=RiStVariUpd
  Data Store Read1 : DataStoreRead  DataStoreName=RiStDlyUpd
  Data Store Write : DataStoreWrite  DataStoreName=RiStVariUpd
  Data Store Write1 : DataStoreWrite  DataStoreName=RiStDlyUpd
  Data Store Write3 : DataStoreWrite  DataStoreName=dWhlImbRejctnLMSqdOutRi
  LimDyn_f32 : NxtrLim/LimDyn_f32
  Product3 : Product  RndMeth=Nearest
  Product5 : Product  Inputs=3
  Product6 : Product  RndMeth=Nearest
  Product7 : Product
  Sum3 : Sum  Inputs=|++
  Sum4 : Sum  Inputs=+
  Unary Minus : UnaryMinus
  output : Outport
  wires:
  Enable/1 -> [enable]
  Constant2/1 -> Product5/1
  PrevEpsilon/1 -> Product5/3  "eps_k-1"
  AdaptiveMu/1 -> Product5/2
  Product5/1 -> Product3/2
  Product6/1 -> Sum3/1
  Product7/1 -> Sum4/1
  [enable] -> Product3/1
  Product3/1 -> Product6/1  "Multiplier"
  x Ref/1 -> Data Store Write1/1, Product7/2  "x_k"
  Constant4/1 -> Unary Minus/1, LimDyn_f32/3
  Unary Minus/1 -> LimDyn_f32/2
  Sum4/1 -> LimDyn_f32/1
  Data Store Read1/1 -> Product6/2  "x_k-1"
  Sum3/1 -> Data Store Write/1, Product7/1  "W_k- xRefStaeVar"
  Data Store Read/1 -> Sum3/2  "x_k-1"
  LimDyn_f32/1 -> Data Store Write3/1, output/1

== system SF015A_WhlImbRejctn/WhlImbRejctn/WhlImbRejctnPer1/Active Rejection Command /Amplitude Calculation ==
  Input : Inport
  Abslt_f32_f32 : NxtrAbslt/Abslt_f32_f32  SFunctionSpec=single y1 = Abslt_f32_f32(single u1)
      settings: AttributesFormatString=%<Name>
  Constant : Constant  Value=ARCHGLBPRM_PIOVER2_ULS_F32
  FilLpUpdOutp : Fil/FilLpUpdOutp  StVar=CmdMgnLp1Fil
      settings: AttributesFormatString=StVar: %<StVar>
  FilLpUpdOutp1 : Fil/FilLpUpdOutp  StVar=CmdMgnLp2Fil
      settings: AttributesFormatString=StVar: %<StVar>
  Product : Product
  Amp : Outport
  wires:
  FilLpUpdOutp1/1 -> Amp/1
  Abslt_f32_f32/1 -> FilLpUpdOutp/1
  Product/1 -> FilLpUpdOutp1/1
  FilLpUpdOutp/1 -> Product/1
  Input/1 -> Abslt_f32_f32/1
  Constant/1 -> Product/2

== system SF015A_WhlImbRejctn/WhlImbRejctn/WhlImbRejctnPer1/Active Rejection Command /CopyRight2 ==

== system SF015A_WhlImbRejctn/WhlImbRejctn/WhlImbRejctnPer1/Active Rejection Command /Phase Adjust - Floating Point ==
  Input Signal : Inport
  Signal Frequency [Hz] : Inport  Port=2
  Abslt_f32_f32 : NxtrAbslt/Abslt_f32_f32  SFunctionSpec=single y1 = Abslt_f32_f32(single u1)
      settings: AttributesFormatString=%<Name>
  Calc Filter Coefficients : Subsystem
  Constant : Constant  Value=ONEHALF_ULS_F32
  Constant1 : Constant  Value=NINETY_ULS_F32
  Filter 1 : Subsystem
  Filter 2 : Subsystem
  FixdToFloat_f32_s16 : FixdToFloat/FixdToFloat_f32_s16  Param1=7
  FloatToFixd_u16_f32 : FloatToFixd/FloatToFixd_u16_f32  Param1=0
  If : If  IfExpression=u1
  If Action Subsystem : Subsystem  TreatAsAtomicUnit=on
  If Action Subsystem1 : Subsystem  TreatAsAtomicUnit=on
  LnrIntrpn_s16_u16VariXs16VariY : LnrIntrpn/LnrIntrpn_s16_u16VariXs16VariY  XTbl=WhlImbRejctnPhaAdjX  YTbl=WhlImbRejctnPhaAdjY
      settings: AttributesFormatString=Lnr ( u16VariX , s16VariY )
  Merge1 : Merge
  Merge2 : Merge
  Product : Product
  Relational Operator : RelationalOperator  Operator=>  OutDataTypeStr=boolean
  Adjusted Signal : Outport
  wires:
  Filter 2/1(Out1) -> Adjusted Signal/1
  Filter 1/1(Out1) -> Filter 2/1(In1)
  [inv_M] -> Filter 2/5(1/Mag)
  [b_0] -> Filter 2/4(b_0)
  [p_k] -> Filter 2/3(p_k)
  [z_m] -> Filter 2/2(z_m)
  [inv_M] -> Filter 1/5(1/Mag)
  [b_0] -> Filter 1/4(b_0)
  [p_k] -> Filter 1/3(p_k)
  [z_m] -> Filter 1/2(z_m)
  Calc Filter Coefficients/4(1/Mag) -> [inv_M]
  Calc Filter Coefficients/2(p_k) -> [p_k]
  Calc Filter Coefficients/1(z_m) -> [z_m]
  Calc Filter Coefficients/3(b_0) -> [b_0]
  FixdToFloat_f32_s16/1 -> If Action Subsystem1/1(Pha_input), If Action Subsystem/1(Pha_input), Abslt_f32_f32/1
  Input Signal/1 -> [PhaseInput]
  FloatToFixd_u16_f32/1 -> LnrIntrpn_s16_u16VariXs16VariY/1
  Relational Operator/1 -> If/1
  If/1 -> If Action Subsystem/Action
  [PhaseInput] -> If Action Subsystem/2(PhaseInput)
  Merge2/1 -> [FinalPhaInput]
  Merge1/1 -> Product/1
  If/2 -> If Action Subsystem1/Action
  [PhaseInput] -> If Action Subsystem1/2(PhaseInput)
  If Action Subsystem/1(Phase) -> Merge1/1
  If Action Subsystem1/1(Phase) -> Merge1/2
  If Action Subsystem/2(FinalPhaInput) -> Merge2/1
  If Action Subsystem1/2(FinalPhaInput) -> Merge2/2
  Signal Frequency [Hz]/1 -> Calc Filter Coefficients/2(freq), FloatToFixd_u16_f32/1
  [FinalPhaInput] -> Filter 1/1(In1)
  Product/1 -> Calc Filter Coefficients/1(phase)
  Constant/1 -> Product/2
  Abslt_f32_f32/1 -> Relational Operator/1
  Constant1/1 -> Relational Operator/2
  LnrIntrpn_s16_u16VariXs16VariY/1 -> FixdToFloat_f32_s16/1
